simulink model "MyModel_Open_v1_1"  (R2018b)
settings: Solver=ode23tb  StartTime=0.0  StopTime=0.5  RelTol=1e-3
InitFcn:
  | Udc1 = 100;
  | Udc2 = 100;
  | tpwm = 1e-4;
  | Td = 0;
libraries: powerlib x33, powerlib_meascontrol x24, powerlib_extras x5, simulink x2
(part 1 of 2)
settings Model: Creator=chenhao  LastModifiedBy=chenhao

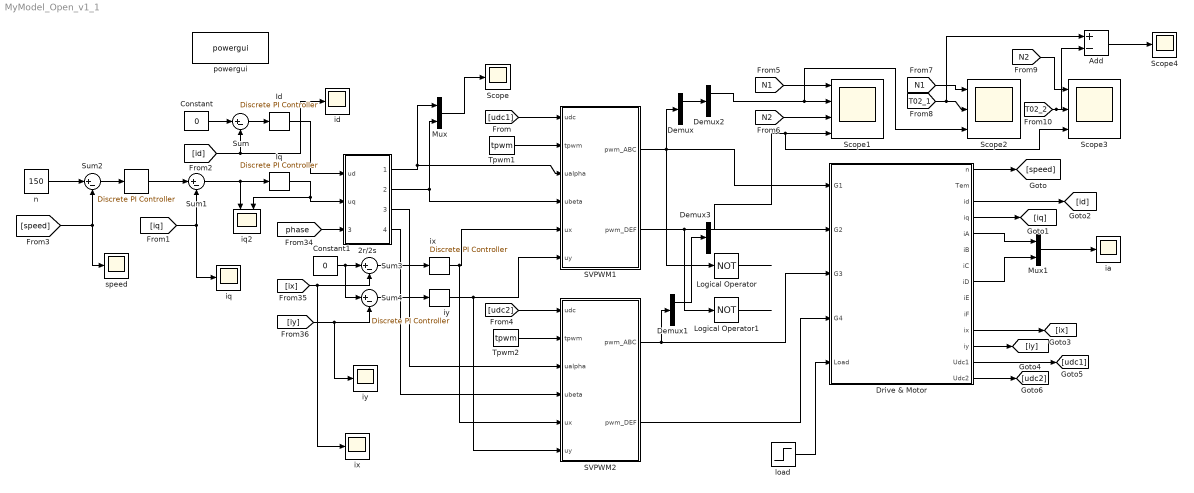
== system MyModel_Open_v1_1 ==
  "    " : powerlib_extras/Discrete  Control Blocks/Discrete PI Controller  Kp=1  Ki=80  Par_Limits=[50 -50]  Init=0  Ts=tpwm
  " Id" : powerlib_extras/Discrete  Control Blocks/Discrete PI Controller  Kp=3  Ki=120  Par_Limits=[300 -300]  Init=0  Ts=tpwm
  " Iq" : powerlib_extras/Discrete  Control Blocks/Discrete PI Controller  Kp=3  Ki=120  Par_Limits=[300 -300]  Init=0  Ts=tpwm
  " ix" : powerlib_extras/Discrete  Control Blocks/Discrete PI Controller  Kp=10  Ki=100  Par_Limits=[300 -300]  Init=0  Ts=tpwm
  " iy" : powerlib_extras/Discrete  Control Blocks/Discrete PI Controller  Kp=10  Ki=100  Par_Limits=[300 -300]  Init=0  Ts=tpwm
  2r/2s : Subsystem
  Add : Sum  Inputs=+-
  Constant : Constant  Value=0
  Constant1 : Constant  Value=0
  Demux : Demux  Outputs=3
  Demux1 : Demux  Outputs=3
  Demux2 : Demux  Outputs=2
  Demux3 : Demux  Outputs=2
  Drive & Motor : Subsystem
  Logical Operator : Logic  Operator=NOT  AllPortsSameDT=off  OutDataTypeStr=boolean
  Logical Operator1 : Logic  Operator=NOT  AllPortsSameDT=off  OutDataTypeStr=boolean
  Mux : Mux  Inputs=2
  Mux1 : Mux  Inputs=2
  SVPWM1 : Subsystem
  SVPWM2 : Subsystem
  Scope : Scope
  Scope1 : Scope  NumInputPorts=4
  Scope2 : Scope  NumInputPorts=3
  Scope3 : Scope  NumInputPorts=3
  Scope4 : Scope
  Sum{,1..4} (5 alike) : Sum  Inputs=|+-
  Tpwm1 : Constant  Value=tpwm
  Tpwm2 : Constant  Value=tpwm
  "ia " : Scope
  "id " : Scope
  iq : Scope
  iq2 : Scope  NumInputPorts=2
  ix : Scope
  iy : Scope
  load : Step  Time=0  After=15  SampleTime=0
  n : Constant  Value=150
  powergui : powerlib/powergui  Priority=1  SimulationMode=Discrete  SampleTime=5e-7  frequency=60  Iterations=50  frequencyindice=0  Pbase=100e6  ErrMax=1e-4  UnitsV=kV  UnitsW=MW  buscounter=0  FunctionMessages=off  echomessages=off  EnableUseOfTLC=off  CurrentSourceSwitches=off  DisableSnubberDevices=off  DisableRonSwitches=off  DisableVfSwitches=off  DisplayEquations=off  SolverType=Tustin/Backward Euler (TBE)  Interpol=off  ExternalGateDelay=off  methode=off  Ts=100  x0status=blocks  SPID=off  SwTol=0  HookPort=off  RestoreLinks=warning  ResistiveCurrentMeasurement=off  Frange=[0:2:500]  Ylog=off  Xlog=on  ShowGrid=off  save=off  variable=ZData  structure=Ia  ZoomFFT=on  StartTime=0.1  cycles=2  DisplayStyle=1  fundamental=2.5  FreqAxis=on  MaxFrequency=30  frequencyindicesteady=1  RmsSteady=1  display=off
  "speed " : Scope
  wires:
  2r/2s/2(ubeta1) -> SVPWM1/4(ubeta), Mux/2
  " ix"/1 -> SVPWM2/5(ux), SVPWM1/5(ux)
  Mux/1 -> Scope/1
  Tpwm1/1 -> SVPWM1/2(tpwm)
  load/1 -> Drive & Motor/5(Load)
  [iy] -> iy/1, Sum4/2
  [iq] -> iq/1, Sum1/2
  Sum3/1 -> " ix"/1
  [udc1] -> SVPWM1/1(udc)
  Sum2/1 -> "    "/1
  2r/2s/1(ualfa1) -> Mux/1, SVPWM1/3(ualpha)
  Sum1/1 -> iq2/1, " Iq"/1
  [speed] -> "speed "/1, Sum2/2
  Sum4/1 -> " iy"/1
  n/1 -> Sum2/1
  [ix] -> ix/1, Sum3/2
  " Id"/1 -> 2r/2s/1(ud)
  [phase] -> 2r/2s/3(theta)
  " Iq"/1 -> iq2/2, 2r/2s/2(uq)
  Sum/1 -> " Id"/1
  Constant1/1 -> Sum4/1, Sum3/1
  "    "/1 -> Sum1/1
  " iy"/1 -> SVPWM2/6(uy), SVPWM1/6(uy)
  [id] -> "id "/1, Sum/2
  Constant/1 -> Sum/1
  Drive & Motor/1(n) -> [speed]
  Drive & Motor/4(iq) -> [iq]
  Drive & Motor/3(id) -> [id]
  Drive & Motor/11(ix) -> [ix]
  Drive & Motor/12(iy) -> [iy]
  Drive & Motor/13(Udc1) -> [udc1]
  Drive & Motor/14(Udc2) -> [udc2]
  Drive & Motor/5(iA) -> Mux1/1
  Drive & Motor/8(iD) -> Mux1/2
  Mux1/1 -> "ia "/1
  [udc2] -> SVPWM2/1(udc)
  Tpwm2/1 -> SVPWM2/2(tpwm)
  2r/2s/3(ualfa2) -> SVPWM2/3(ualpha)
  2r/2s/4(ubeta2) -> SVPWM2/4(ubeta)
  SVPWM1/1(pwm_ABC) -> Demux/1, Logical Operator/1, Drive & Motor/1(G1)
  SVPWM1/2(pwm_DEF) -> Logical Operator1/1, Drive & Motor/2(G2)
  Logical Operator/1 -> ?
  SVPWM2/1(pwm_ABC) -> Demux1/1, Drive & Motor/3(G3)
  SVPWM2/2(pwm_DEF) -> Drive & Motor/4(G4)
  Logical Operator1/1 -> ?
  [N1] -> Scope1/1
  [N2] -> Scope1/3
  Demux/1 -> Demux2/1
  Demux2/1 -> Scope2/3, Scope1/2
  Demux1/1 -> Demux3/1
  Demux3/1 -> Scope3/3, Scope1/4
  [N1] -> Scope2/1
  [T02_1] -> Add/1, Scope2/2
  [N2] -> Scope3/1
  [T02_2] -> Add/2, Scope3/2
  Add/1 -> Scope4/1

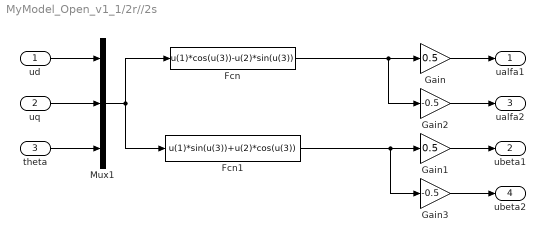
== system MyModel_Open_v1_1/2r//2s ==
  ud : Inport
  uq : Inport  Port=2
  theta : Inport  Port=3
  Fcn : Fcn  Expr=u(1)*cos(u(3))-u(2)*sin(u(3))
  Fcn1 : Fcn  Expr=u(1)*sin(u(3))+u(2)*cos(u(3))
  Gain : Gain  Gain=0.5
  Gain1 : Gain  Gain=0.5
  Gain2 : Gain  Gain=-0.5
  Gain3 : Gain  Gain=-0.5
  Mux1 : Mux  Inputs=3
  ualfa1 : Outport
  ubeta1 : Outport  Port=2
  ualfa2 : Outport  Port=3
  ubeta2 : Outport  Port=4
  wires:
  theta/1 -> Mux1/3
  uq/1 -> Mux1/2
  ud/1 -> Mux1/1
  Mux1/1 -> Fcn1/1, Fcn/1
  Fcn/1 -> Gain2/1, Gain/1
  Gain/1 -> ualfa1/1
  Gain1/1 -> ubeta1/1
  Fcn1/1 -> Gain3/1, Gain1/1
  Gain2/1 -> ualfa2/1
  Gain3/1 -> ubeta2/1

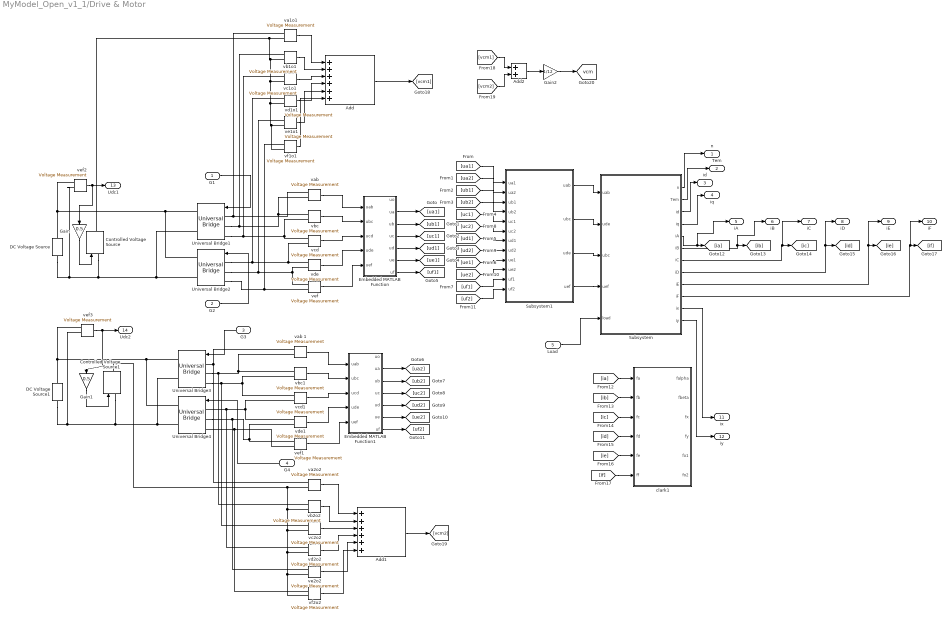
== system MyModel_Open_v1_1/Drive & Motor ==
  G1 : Inport
  G2 : Inport  Port=2
  G3 : Inport  Port=3
  G4 : Inport  Port=4
  Load : Inport  Port=5
  Add : Sum  Inputs=++++++
  Add1 : Sum  Inputs=++++++
  Add2 : Sum
  Controlled Voltage Source : powerlib/Electrical Sources/Controlled Voltage Source  Initialize=on  Source_Type=AC  Amplitude=0  Phase=0  Frequency=0  Measurements=None
  Controlled Voltage Source1 : powerlib/Electrical Sources/Controlled Voltage Source  Initialize=on  Source_Type=AC  Amplitude=0  Phase=0  Frequency=0  Measurements=None
  DC Voltage Source : powerlib/Electrical Sources/DC Voltage Source  Amplitude=Udc1  Measurements=Voltage
  DC Voltage Source1 : powerlib/Electrical Sources/DC Voltage Source  Amplitude=Udc2  Measurements=Voltage
  Embedded MATLAB Function : MATLAB Function  TreatAsAtomicUnit=on
  Embedded MATLAB Function1 : MATLAB Function  TreatAsAtomicUnit=on
  Gain : Gain  Gain=0.5
  Gain1 : Gain  Gain=0.5
  Gain2 : Gain  Gain=1/12
  Subsystem : Subsystem
  Subsystem1 : Subsystem
  Universal Bridge{1..4} (4 alike) : powerlib/Power Electronics/Universal Bridge  Arms=3  SnubberResistance=1e5  SnubberCapacitance=inf  Device=IGBT / Diodes  Ron=1e-3  Lon=0  ForwardVoltages="[  0  0  ]"  ForwardVoltage=0  GTOparameters=[ 10e-6 , 20e-6 ]  IGBTparameters=[ 0 , 0 ]  Measurements=None  Measurements_2=None  converterType=Rectifier
  clark1 : MATLAB Function  TreatAsAtomicUnit=on
  va1o1 : powerlib/Measurements/Voltage Measurement  PhasorSimulation=off  OutputType=Complex  PSBequivalent=0
  va2o2 : powerlib/Measurements/Voltage Measurement  PhasorSimulation=off  OutputType=Complex  PSBequivalent=0
  "vab " : powerlib/Measurements/Voltage Measurement  PhasorSimulation=off  OutputType=Complex  PSBequivalent=0
  vab 1 : powerlib/Measurements/Voltage Measurement  PhasorSimulation=off  OutputType=Complex  PSBequivalent=0
  vb1o1 : powerlib/Measurements/Voltage Measurement  PhasorSimulation=off  OutputType=Complex  PSBequivalent=0
  vb2o2 : powerlib/Measurements/Voltage Measurement  PhasorSimulation=off  OutputType=Complex  PSBequivalent=0
  vbc : powerlib/Measurements/Voltage Measurement  PhasorSimulation=off  OutputType=Complex  PSBequivalent=0
  vbc1 : powerlib/Measurements/Voltage Measurement  PhasorSimulation=off  OutputType=Complex  PSBequivalent=0
  vc1o1 : powerlib/Measurements/Voltage Measurement  PhasorSimulation=off  OutputType=Complex  PSBequivalent=0
  vc2o2 : powerlib/Measurements/Voltage Measurement  PhasorSimulation=off  OutputType=Complex  PSBequivalent=0
  vcd : powerlib/Measurements/Voltage Measurement  PhasorSimulation=off  OutputType=Complex  PSBequivalent=0
  vcd1 : powerlib/Measurements/Voltage Measurement  PhasorSimulation=off  OutputType=Complex  PSBequivalent=0
  vd1o1 : powerlib/Measurements/Voltage Measurement  PhasorSimulation=off  OutputType=Complex  PSBequivalent=0
  vd2o2 : powerlib/Measurements/Voltage Measurement  PhasorSimulation=off  OutputType=Complex  PSBequivalent=0
  vde : powerlib/Measurements/Voltage Measurement  PhasorSimulation=off  OutputType=Complex  PSBequivalent=0
  vde1 : powerlib/Measurements/Voltage Measurement  PhasorSimulation=off  OutputType=Complex  PSBequivalent=0
  ve1o1 : powerlib/Measurements/Voltage Measurement  PhasorSimulation=off  OutputType=Complex  PSBequivalent=0
  ve2o2 : powerlib/Measurements/Voltage Measurement  PhasorSimulation=off  OutputType=Complex  PSBequivalent=0
  vef{,1..3} (4 alike) : powerlib/Measurements/Voltage Measurement  PhasorSimulation=off  OutputType=Complex  PSBequivalent=0
  vf1o1 : powerlib/Measurements/Voltage Measurement  PhasorSimulation=off  OutputType=Complex  PSBequivalent=0
  vf2o2 : powerlib/Measurements/Voltage Measurement  PhasorSimulation=off  OutputType=Complex  PSBequivalent=0
  n : Outport
  Tem : Outport  Port=2
  id : Outport  Port=3
  iq : Outport  Port=4
  iA : Outport  Port=5
  iB : Outport  Port=6
  iC : Outport  Port=7
  iD : Outport  Port=8
  iE : Outport  Port=9
  iF : Outport  Port=10
  ix : Outport  Port=11
  iy : Outport  Port=12
  Udc1 : Outport  Port=13
  Udc2 : Outport  Port=14
  tag scope: vcm=global
  wires:
  G1/1 -> Universal Bridge1/1
  G2/1 -> Universal Bridge2/1
  G3/1 -> Universal Bridge3/1
  G4/1 -> Universal Bridge4/1
  vef/1 -> Embedded MATLAB Function/5(uef)
  vde/1 -> Embedded MATLAB Function/4(ude)
  "vab "/1 -> Embedded MATLAB Function/1(uab)
  vcd/1 -> Embedded MATLAB Function/3(ucd)
  vbc/1 -> Embedded MATLAB Function/2(ubc)
  Embedded MATLAB Function/2(ua) -> [ua1]
  Embedded MATLAB Function/3(ub) -> [ub1]
  Embedded MATLAB Function/4(uc) -> [uc1]
  Embedded MATLAB Function/5(ud) -> [ud1]
  Embedded MATLAB Function/6(ue) -> [ue1]
  Embedded MATLAB Function/7(uf) -> [uf1]
  Embedded MATLAB Function1/2(ua) -> [ua2]
  Embedded MATLAB Function1/3(ub) -> [ub2]
  Embedded MATLAB Function1/4(uc) -> [uc2]
  Embedded MATLAB Function1/5(ud) -> [ud2]
  Embedded MATLAB Function1/6(ue) -> [ue2]
  Embedded MATLAB Function1/7(uf) -> [uf2]
  vab 1/1 -> Embedded MATLAB Function1/1(uab)
  vbc1/1 -> Embedded MATLAB Function1/2(ubc)
  vcd1/1 -> Embedded MATLAB Function1/3(ucd)
  vde1/1 -> Embedded MATLAB Function1/4(ude)
  vef1/1 -> Embedded MATLAB Function1/5(uef)
  [ua1] -> Subsystem1/1(ua1)
  [ua2] -> Subsystem1/2(ua2)
  [ub1] -> Subsystem1/3(ub1)
  [ub2] -> Subsystem1/4(ub2)
  [uc1] -> Subsystem1/5(uc1)
  [uc2] -> Subsystem1/6(uc2)
  [ud1] -> Subsystem1/7(ud1)
  [ud2] -> Subsystem1/8(ud2)
  [ue1] -> Subsystem1/9(ue1)
  [ue2] -> Subsystem1/10(ue2)
  [uf1] -> Subsystem1/11(uf1)
  [uf2] -> Subsystem1/12(uf2)
  Load/1 -> Subsystem/5(load)
  Subsystem/1(n) -> n/1
  Subsystem/2(Tem) -> Tem/1
  Subsystem/3(id) -> id/1
  Subsystem/4(iq) -> iq/1
  Subsystem/5(iA) -> iA/1, [ia]
  Subsystem/6(iB) -> iB/1, [ib]
  Subsystem/7(iC) -> iC/1, [ic]
  Subsystem/8(iD) -> iD/1, [id]
  Subsystem/9(iE) -> iE/1, [ie]
  Subsystem/10(iF) -> iF/1, [if]
  [ia] -> clark1/1(fa)
  [ib] -> clark1/2(fb)
  [ic] -> clark1/3(fc)
  [id] -> clark1/4(fd)
  [ie] -> clark1/5(fe)
  [if] -> clark1/6(ff)
  vef2/1 -> Udc1/1, Gain/1
  vef3/1 -> Gain1/1, Udc2/1
  Gain/1 -> Controlled Voltage Source/1
  Gain1/1 -> Controlled Voltage Source1/1
  va1o1/1 -> Add/1
  vb1o1/1 -> Add/2
  vc1o1/1 -> Add/3
  vd1o1/1 -> Add/4
  ve1o1/1 -> Add/5
  vf1o1/1 -> Add/6
  Add/1 -> [vcm1]
  va2o2/1 -> Add1/1
  vb2o2/1 -> Add1/2
  vc2o2/1 -> Add1/3
  vd2o2/1 -> Add1/4
  ve2o2/1 -> Add1/5
  vf2o2/1 -> Add1/6
  Add1/1 -> [vcm2]
  [vcm1] -> Add2/1
  [vcm2] -> Add2/2
  Add2/1 -> Gain2/1
  Gain2/1 -> [vcm]
  Subsystem1/4(uef) -> Subsystem/4(uef)
  Subsystem1/3(ude) -> Subsystem/3(ubc)
  Subsystem1/2(ubc) -> Subsystem/2(ude)
  Subsystem1/1(uab) -> Subsystem/1(uab)
  Subsystem/11(ix) -> ix/1
  Subsystem/12(iy) -> iy/1
  connections:
  vde1/LConn1 -- vcd1/LConn2 -- vd2o2/LConn1 -- Universal Bridge4/LConn1
  vde/LConn1 -- vd1o1/LConn1 -- Universal Bridge2/LConn1 -- vcd/LConn2
  vef1/LConn2 -- Universal Bridge4/LConn3 -- vf2o2/LConn1
  Universal Bridge1/RConn2 -- Controlled Voltage Source/LConn1 -- vef2/LConn2 -- DC Voltage Source/LConn1 -- Universal Bridge2/RConn2
  DC Voltage Source/RConn1 -- Universal Bridge2/RConn1 -- Universal Bridge1/RConn1 -- vef2/LConn1
  Universal Bridge3/LConn1 -- vab 1/LConn1 -- va2o2/LConn1
  vbc/LConn1 -- vb1o1/LConn1 -- Universal Bridge1/LConn2 -- "vab "/LConn2
  vbc1/LConn1 -- vb2o2/LConn1 -- Universal Bridge3/LConn2 -- vab 1/LConn2
  vcd/LConn1 -- vc1o1/LConn1 -- Universal Bridge1/LConn3 -- vbc/LConn2
  vbc1/LConn2 -- vc2o2/LConn1 -- Universal Bridge3/LConn3 -- vcd1/LConn1
  Universal Bridge3/RConn1 -- vef3/LConn1 -- DC Voltage Source1/RConn1 -- Universal Bridge4/RConn1
  Universal Bridge3/RConn2 -- vef3/LConn2 -- DC Voltage Source1/LConn1 -- Controlled Voltage Source1/LConn1 -- Universal Bridge4/RConn2
  vef1/LConn1 -- ve2o2/LConn1 -- Universal Bridge4/LConn2 -- vde1/LConn2
  Universal Bridge1/LConn1 -- "vab "/LConn1 -- va1o1/LConn1
  vef/LConn1 -- ve1o1/LConn1 -- Universal Bridge2/LConn2 -- vde/LConn2
  Universal Bridge2/LConn3 -- vf1o1/LConn1 -- vef/LConn2
  va1o1/LConn2 -- vf1o1/LConn2 -- ve1o1/LConn2 -- vd1o1/LConn2 -- vc1o1/LConn2 -- vb1o1/LConn2 -- Controlled Voltage Source/RConn1
  va2o2/LConn2 -- vf2o2/LConn2 -- ve2o2/LConn2 -- vd2o2/LConn2 -- vc2o2/LConn2 -- vb2o2/LConn2 -- Controlled Voltage Source1/RConn1

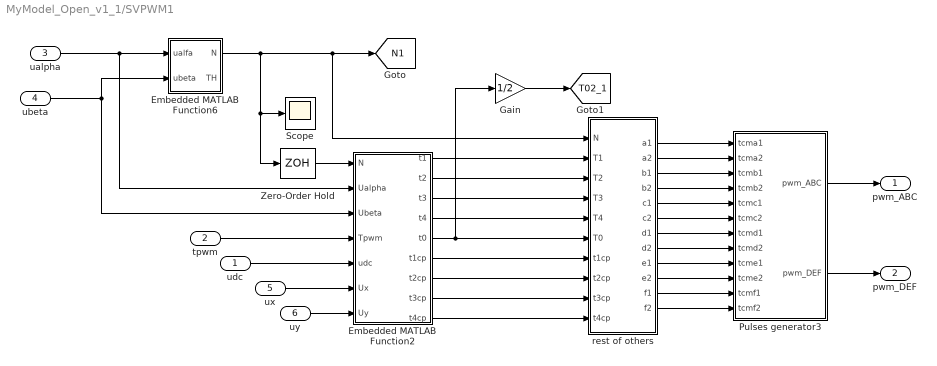
== system MyModel_Open_v1_1/SVPWM1 ==
  udc : Inport
  tpwm : Inport  Port=2
  ualpha : Inport  Port=3
  ubeta : Inport  Port=4
  ux : Inport  Port=5
  uy : Inport  Port=6
  Embedded MATLAB Function2 : MATLAB Function  TreatAsAtomicUnit=on
  Embedded MATLAB Function6 : MATLAB Function  TreatAsAtomicUnit=on
  Gain : Gain  Gain=1/2
  Pulses generator3 : Subsystem
  Scope : Scope
  Zero-Order Hold : ZeroOrderHold  SampleTime=1e-4
  rest of others : MATLAB Function  TreatAsAtomicUnit=on
  pwm_ABC : Outport
  pwm_DEF : Outport  Port=2
  tag scope: N1=global, T02_1=global
  wires:
  udc/1 -> Embedded MATLAB Function2/5(udc)
  Embedded MATLAB Function2/4(t4) -> rest of others/5(T4)
  Embedded MATLAB Function2/1(t1) -> rest of others/2(T1)
  Pulses generator3/1(pwm_ABC) -> pwm_ABC/1
  Pulses generator3/2(pwm_DEF) -> pwm_DEF/1
  rest of others/12(f2) -> Pulses generator3/12(tcmf2)
  rest of others/11(f1) -> Pulses generator3/11(tcmf1)
  rest of others/10(e2) -> Pulses generator3/10(tcme2)
  rest of others/9(e1) -> Pulses generator3/9(tcme1)
  rest of others/8(d2) -> Pulses generator3/8(tcmd2)
  rest of others/7(d1) -> Pulses generator3/7(tcmd1)
  rest of others/6(c2) -> Pulses generator3/6(tcmc2)
  rest of others/5(c1) -> Pulses generator3/5(tcmc1)
  rest of others/4(b2) -> Pulses generator3/4(tcmb2)
  rest of others/3(b1) -> Pulses generator3/3(tcmb1)
  rest of others/2(a2) -> Pulses generator3/2(tcma2)
  rest of others/1(a1) -> Pulses generator3/1(tcma1)
  Embedded MATLAB Function2/2(t2) -> rest of others/3(T2)
  tpwm/1 -> Embedded MATLAB Function2/4(Tpwm)
  Embedded MATLAB Function2/5(t0) -> Gain/1, rest of others/6(T0)
  ualpha/1 -> Embedded MATLAB Function2/2(Ualpha), Embedded MATLAB Function6/1(ualfa)
  ubeta/1 -> Embedded MATLAB Function6/2(ubeta), Embedded MATLAB Function2/3(Ubeta)
  ux/1 -> Embedded MATLAB Function2/6(Ux)
  uy/1 -> Embedded MATLAB Function2/7(Uy)
  Embedded MATLAB Function2/3(t3) -> rest of others/4(T3)
  Zero-Order Hold/1 -> Embedded MATLAB Function2/1(N)
  Embedded MATLAB Function6/1(N) -> [N1], rest of others/1(N), Scope/1, Zero-Order Hold/1
  Embedded MATLAB Function2/9(t4cp) -> rest of others/10(t4cp)
  Embedded MATLAB Function2/8(t3cp) -> rest of others/9(t3cp)
  Embedded MATLAB Function2/7(t2cp) -> rest of others/8(t2cp)
  Embedded MATLAB Function2/6(t1cp) -> rest of others/7(t1cp)
  Gain/1 -> [T02_1]

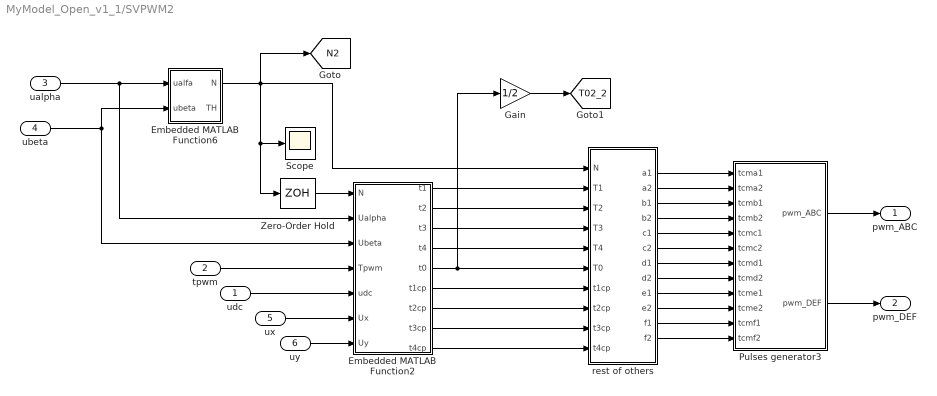
== system MyModel_Open_v1_1/SVPWM2 ==
  udc : Inport
  tpwm : Inport  Port=2
  ualpha : Inport  Port=3
  ubeta : Inport  Port=4
  ux : Inport  Port=5
  uy : Inport  Port=6
  Embedded MATLAB Function2 : MATLAB Function  TreatAsAtomicUnit=on
  Embedded MATLAB Function6 : MATLAB Function  TreatAsAtomicUnit=on
  Gain : Gain  Gain=1/2
  Pulses generator3 : Subsystem
  Scope : Scope
  Zero-Order Hold : ZeroOrderHold  SampleTime=1e-4
  rest of others : MATLAB Function  TreatAsAtomicUnit=on
  pwm_ABC : Outport
  pwm_DEF : Outport  Port=2
  tag scope: N2=global, T02_2=global
  wires:
  Embedded MATLAB Function2/6(t1cp) -> rest of others/7(t1cp)
  Embedded MATLAB Function2/7(t2cp) -> rest of others/8(t2cp)
  Embedded MATLAB Function2/8(t3cp) -> rest of others/9(t3cp)
  Embedded MATLAB Function2/9(t4cp) -> rest of others/10(t4cp)
  Embedded MATLAB Function6/1(N) -> Zero-Order Hold/1, Scope/1, rest of others/1(N), [N2]
  Zero-Order Hold/1 -> Embedded MATLAB Function2/1(N)
  Embedded MATLAB Function2/3(t3) -> rest of others/4(T3)
  uy/1 -> Embedded MATLAB Function2/7(Uy)
  ux/1 -> Embedded MATLAB Function2/6(Ux)
  ubeta/1 -> Embedded MATLAB Function2/3(Ubeta), Embedded MATLAB Function6/2(ubeta)
  ualpha/1 -> Embedded MATLAB Function6/1(ualfa), Embedded MATLAB Function2/2(Ualpha)
  Embedded MATLAB Function2/5(t0) -> Gain/1, rest of others/6(T0)
  tpwm/1 -> Embedded MATLAB Function2/4(Tpwm)
  Embedded MATLAB Function2/2(t2) -> rest of others/3(T2)
  rest of others/1(a1) -> Pulses generator3/1(tcma1)
  rest of others/2(a2) -> Pulses generator3/2(tcma2)
  rest of others/3(b1) -> Pulses generator3/3(tcmb1)
  rest of others/4(b2) -> Pulses generator3/4(tcmb2)
  rest of others/5(c1) -> Pulses generator3/5(tcmc1)
  rest of others/6(c2) -> Pulses generator3/6(tcmc2)
  rest of others/7(d1) -> Pulses generator3/7(tcmd1)
  rest of others/8(d2) -> Pulses generator3/8(tcmd2)
  rest of others/9(e1) -> Pulses generator3/9(tcme1)
  rest of others/10(e2) -> Pulses generator3/10(tcme2)
  rest of others/11(f1) -> Pulses generator3/11(tcmf1)
  rest of others/12(f2) -> Pulses generator3/12(tcmf2)
  Pulses generator3/2(pwm_DEF) -> pwm_DEF/1
  Pulses generator3/1(pwm_ABC) -> pwm_ABC/1
  Embedded MATLAB Function2/1(t1) -> rest of others/2(T1)
  Embedded MATLAB Function2/4(t4) -> rest of others/5(T4)
  udc/1 -> Embedded MATLAB Function2/5(udc)
  Gain/1 -> [T02_2]

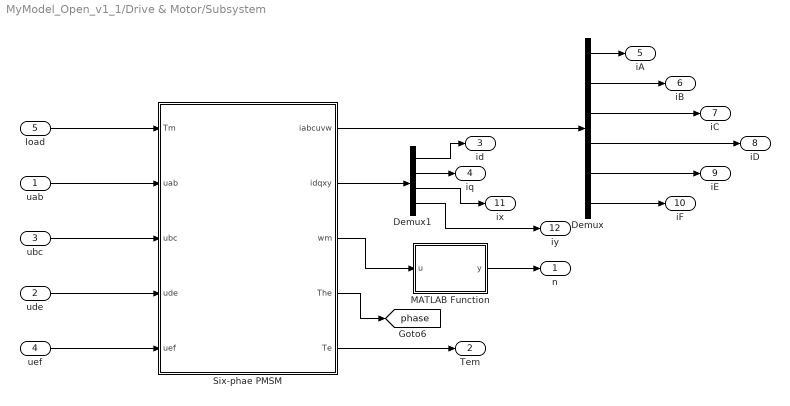
== system MyModel_Open_v1_1/Drive & Motor/Subsystem ==
  uab : Inport
  ude : Inport  Port=2
  ubc : Inport  Port=3
  uef : Inport  Port=4
  load : Inport  Port=5
  Demux : Demux  Outputs=6
  Demux1 : Demux
  MATLAB Function : MATLAB Function  TreatAsAtomicUnit=on
  Six-phae PMSM : Subsystem  mask{R=0.099, Ld=2.463342136542000e-03, Lq=2.473254136542000e-03, Lz=1.520747e-3, Flux=0.0592, J=0.00174, F=0, p=5}
      mask prompts: R "R(ohm)"; Ld "Ld(H)"; Lq "Lq(H)"; Lz "Lz(H)"; Flux "Flux(Wb)"; J "J(kg.m^2)"; F "F(N.m.s)"
  n : Outport
  Tem : Outport  Port=2
  id : Outport  Port=3
  iq : Outport  Port=4
  iA : Outport  Port=5
  iB : Outport  Port=6
  iC : Outport  Port=7
  iD : Outport  Port=8
  iE : Outport  Port=9
  iF : Outport  Port=10
  ix : Outport  Port=11
  iy : Outport  Port=12
  tag scope: phase=global
  wires:
  Demux/6 -> iF/1
  Demux1/2 -> iq/1
  uef/1 -> Six-phae PMSM/5(uef)
  Demux/5 -> iE/1
  Demux/2 -> iB/1
  Demux/1 -> iA/1
  Six-phae PMSM/5(Te) -> Tem/1
  uab/1 -> Six-phae PMSM/2(uab)
  Demux1/1 -> id/1
  ubc/1 -> Six-phae PMSM/3(ubc)
  Demux/3 -> iC/1
  MATLAB Function/1(y) -> n/1
  load/1 -> Six-phae PMSM/1(Tm)
  Demux/4 -> iD/1
  ude/1 -> Six-phae PMSM/4(ude)
  Six-phae PMSM/1(iabcuvw) -> Demux/1
  Six-phae PMSM/2(idqxy) -> Demux1/1
  Demux1/3 -> ix/1
  Demux1/4 -> iy/1
  Six-phae PMSM/3(wm) -> MATLAB Function/1(u)
  Six-phae PMSM/4(The) -> [phase]

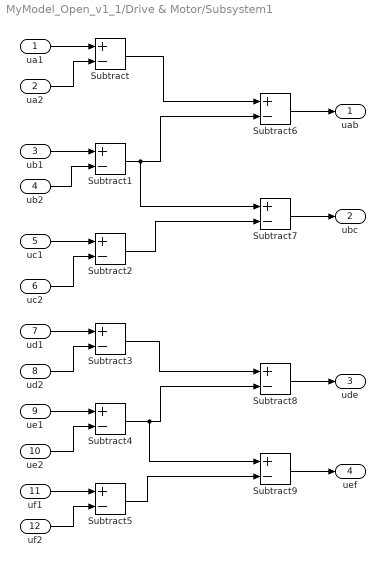
== system MyModel_Open_v1_1/Drive & Motor/Subsystem1 ==
  ua1 : Inport
  ua2 : Inport  Port=2
  ub1 : Inport  Port=3
  ub2 : Inport  Port=4
  uc1 : Inport  Port=5
  uc2 : Inport  Port=6
  ud1 : Inport  Port=7
  ud2 : Inport  Port=8
  ue1 : Inport  Port=9
  ue2 : Inport  Port=10
  uf1 : Inport  Port=11
  uf2 : Inport  Port=12
  Subtract{,1..9} (10 alike) : Sum  Inputs=+-
  uab : Outport
  ubc : Outport  Port=2
  ude : Outport  Port=3
  uef : Outport  Port=4
  wires:
  ua1/1 -> Subtract/1
  ua2/1 -> Subtract/2
  Subtract/1 -> Subtract6/1
  ub1/1 -> Subtract1/1
  ub2/1 -> Subtract1/2
  Subtract1/1 -> Subtract7/1, Subtract6/2
  uc1/1 -> Subtract2/1
  uc2/1 -> Subtract2/2
  Subtract2/1 -> Subtract7/2
  ud1/1 -> Subtract3/1
  ud2/1 -> Subtract3/2
  Subtract3/1 -> Subtract8/1
  ue1/1 -> Subtract4/1
  ue2/1 -> Subtract4/2
  Subtract4/1 -> Subtract9/1, Subtract8/2
  uf1/1 -> Subtract5/1
  uf2/1 -> Subtract5/2
  Subtract5/1 -> Subtract9/2
  Subtract6/1 -> uab/1
  Subtract7/1 -> ubc/1
  Subtract8/1 -> ude/1
  Subtract9/1 -> uef/1

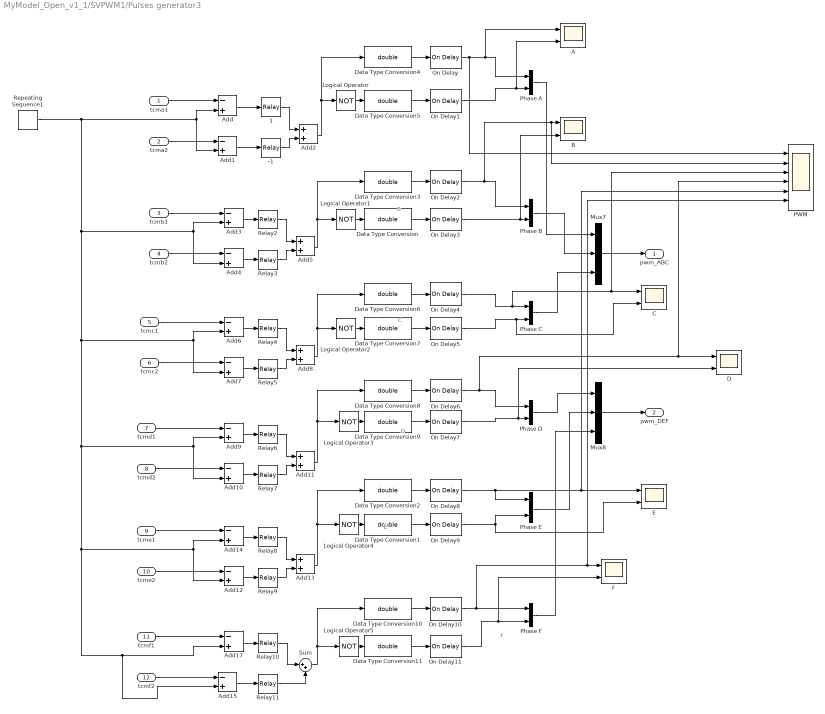
== system MyModel_Open_v1_1/SVPWM1/Pulses generator3 ==
  note: B
  note: C
  note: D
  note: E
  note: F
  tcma1 : Inport
  tcma2 : Inport  Port=2
  tcmb1 : Inport  Port=3
  tcmb2 : Inport  Port=4
  tcmc1 : Inport  Port=5
  tcmc2 : Inport  Port=6
  tcmd1 : Inport  Port=7
  tcmd2 : Inport  Port=8
  tcme1 : Inport  Port=9
  tcme2 : Inport  Port=10
  tcmf1 : Inport  Port=11
  tcmf2 : Inport  Port=12
  -1 : Relay  OnOutputValue=-1
  1 : Relay
  A : Scope  NumInputPorts=2
  Add{,1,3..4,6..7,9..10,12,14..15,17} (12 alike) : Sum  Inputs=-+
  Add{2,5,8,11,13} (5 alike) : Sum
  B : Scope  NumInputPorts=2
  C : Scope  NumInputPorts=2
  D : Scope  NumInputPorts=2
  Data Type Conversion{,1..11} (12 alike) : DataTypeConversion  OutDataTypeStr=double
  E : Scope  NumInputPorts=2
  F : Scope  NumInputPorts=2
  Logical Operator{,1..5} (6 alike) : Logic  Operator=NOT  AllPortsSameDT=off  OutDataTypeStr=boolean
  Mux7 : Mux  Inputs=3
  Mux8 : Mux  Inputs=3
  On Delay{,1..11} (12 alike) : powerlib_meascontrol/Logic/On Delay  DelayType=On delay  delay=Td  ic=0  Ts=0
      settings: SourceProductName=Simscape Power Systems
  PWM : Scope  NumInputPorts=6
  Phase A : Mux  Inputs=2
  Phase B : Mux  Inputs=2
  Phase C : Mux  Inputs=2
  Phase D : Mux  Inputs=2
  Phase E : Mux  Inputs=2
  Phase F : Mux  Inputs=2
  Relay{2,4,6,8,10} (5 alike) : Relay
  Relay{3,5,7,9,11} (5 alike) : Relay  OnOutputValue=-1
  Repeating Sequence1 : simulink/Sources/Repeating Sequence  rep_seq_t=[0 tpwm]  rep_seq_y=[0 tpwm]
  Sum : Sum  Inputs=|++
  pwm_ABC : Outport
  pwm_DEF : Outport  Port=2
  wires:
  On Delay11/1 -> F/2, Phase F/2
  Data Type Conversion11/1 -> On Delay11/1
  On Delay10/1 -> PWM/6, F/1, Phase F/1
  Data Type Conversion10/1 -> On Delay10/1
  On Delay9/1 -> E/2, Phase E/2
  Data Type Conversion1/1 -> On Delay9/1
  On Delay8/1 -> Phase E/1, PWM/5, E/1
  Data Type Conversion2/1 -> On Delay8/1
  On Delay7/1 -> D/2, Phase D/2
  Data Type Conversion9/1 -> On Delay7/1
  On Delay6/1 -> PWM/4, D/1, Phase D/1
  Data Type Conversion8/1 -> On Delay6/1
  On Delay5/1 -> C/2, Phase C/2
  Data Type Conversion7/1 -> On Delay5/1
  On Delay4/1 -> PWM/3, C/1, Phase C/1
  Data Type Conversion6/1 -> On Delay4/1
  On Delay2/1 -> PWM/2, B/1, Phase B/1
  On Delay3/1 -> B/2, Phase B/2
  Data Type Conversion/1 -> On Delay3/1
  Data Type Conversion3/1 -> On Delay2/1
  On Delay1/1 -> A/2, Phase A/2
  Data Type Conversion5/1 -> On Delay1/1
  On Delay/1 -> A/1, Phase A/1, PWM/1
  Data Type Conversion4/1 -> On Delay/1
  Logical Operator3/1 -> Data Type Conversion9/1
  Logical Operator2/1 -> Data Type Conversion7/1
  Logical Operator/1 -> Data Type Conversion5/1
  Logical Operator1/1 -> Data Type Conversion/1
  Logical Operator4/1 -> Data Type Conversion1/1
  Add5/1 -> Logical Operator1/1, Data Type Conversion3/1
  Add2/1 -> Logical Operator/1, Data Type Conversion4/1
  Mux8/1 -> pwm_DEF/1
  Mux7/1 -> pwm_ABC/1
  Sum/1 -> Logical Operator5/1, Data Type Conversion10/1
  Add13/1 -> Logical Operator4/1, Data Type Conversion2/1
  Add11/1 -> Logical Operator3/1, Data Type Conversion8/1
  Add8/1 -> Logical Operator2/1, Data Type Conversion6/1
  Logical Operator5/1 -> Data Type Conversion11/1
  tcmf2/1 -> Add15/1
  Relay11/1 -> Sum/2
  Relay10/1 -> Sum/1
  Add17/1 -> Relay10/1
  tcmf1/1 -> Add17/1
  tcme2/1 -> Add12/1
  Relay9/1 -> Add13/2
  Relay8/1 -> Add13/1
  Add12/1 -> Relay9/1
  Add14/1 -> Relay8/1
  tcme1/1 -> Add14/1
  tcmd2/1 -> Add10/1
  Relay7/1 -> Add11/2
  Relay6/1 -> Add11/1
  Add10/1 -> Relay7/1
  Add9/1 -> Relay6/1
  tcmd1/1 -> Add9/1
  tcmc2/1 -> Add7/1
  Relay5/1 -> Add8/2
  Relay4/1 -> Add8/1
  Add7/1 -> Relay5/1
  Add6/1 -> Relay4/1
  tcmb2/1 -> Add4/1
  Relay3/1 -> Add5/2
  Relay2/1 -> Add5/1
  Add4/1 -> Relay3/1
  Add3/1 -> Relay2/1
  tcma1/1 -> Add/1
  -1/1 -> Add2/2
  1/1 -> Add2/1
  Add1/1 -> -1/1
  Add/1 -> 1/1
  Repeating Sequence1/1 -> Add15/2, Add17/2, Add12/2, Add14/2, Add9/2, Add10/2, Add7/2, Add6/2, Add3/2, Add4/2, Add1/2, Add/2
  tcma2/1 -> Add1/1
  tcmb1/1 -> Add3/1
  tcmc1/1 -> Add6/1
  Add15/1 -> Relay11/1
  Phase A/1 -> Mux7/1
  Phase B/1 -> Mux7/2
  Phase C/1 -> Mux7/3
  Phase D/1 -> Mux8/1
  Phase E/1 -> Mux8/2
  Phase F/1 -> Mux8/3

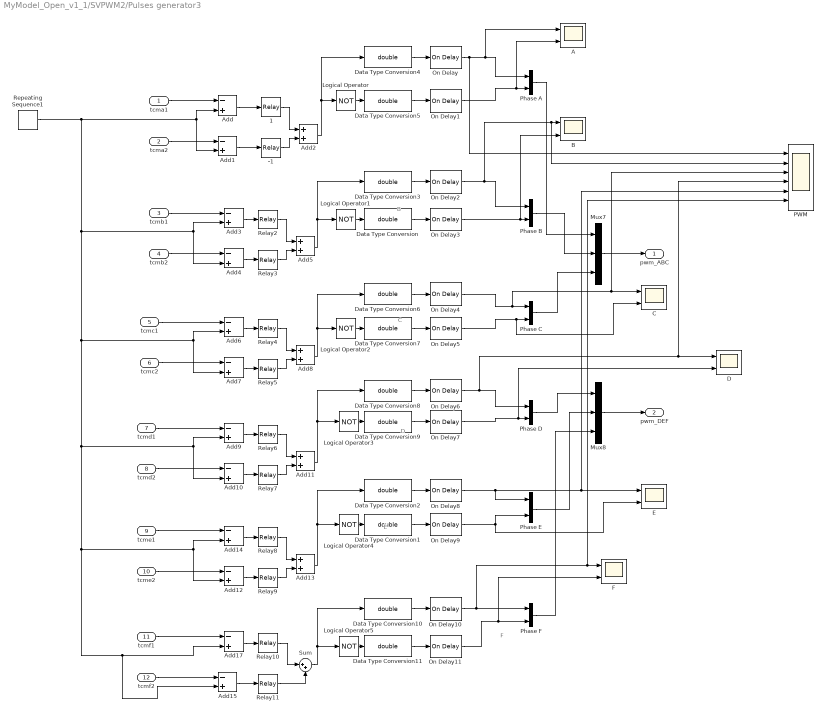
== system MyModel_Open_v1_1/SVPWM2/Pulses generator3 ==
  note: F
  note: E
  note: D
  note: C
  note: B
  tcma1 : Inport
  tcma2 : Inport  Port=2
  tcmb1 : Inport  Port=3
  tcmb2 : Inport  Port=4
  tcmc1 : Inport  Port=5
  tcmc2 : Inport  Port=6
  tcmd1 : Inport  Port=7
  tcmd2 : Inport  Port=8
  tcme1 : Inport  Port=9
  tcme2 : Inport  Port=10
  tcmf1 : Inport  Port=11
  tcmf2 : Inport  Port=12
  -1 : Relay  OnOutputValue=-1
  1 : Relay
  A : Scope  NumInputPorts=2
  Add{,1,3..4,6..7,9..10,12,14..15,17} (12 alike) : Sum  Inputs=-+
  Add{2,5,8,11,13} (5 alike) : Sum
  B : Scope  NumInputPorts=2
  C : Scope  NumInputPorts=2
  D : Scope  NumInputPorts=2
  Data Type Conversion{,1..11} (12 alike) : DataTypeConversion  OutDataTypeStr=double
  E : Scope  NumInputPorts=2
  F : Scope  NumInputPorts=2
  Logical Operator{,1..5} (6 alike) : Logic  Operator=NOT  AllPortsSameDT=off  OutDataTypeStr=boolean
  Mux7 : Mux  Inputs=3
  Mux8 : Mux  Inputs=3
  On Delay{,1..11} (12 alike) : powerlib_meascontrol/Logic/On Delay  DelayType=On delay  delay=Td  ic=0  Ts=0
      settings: SourceProductName=Simscape Power Systems
  PWM : Scope  NumInputPorts=6
  Phase A : Mux  Inputs=2
  Phase B : Mux  Inputs=2
  Phase C : Mux  Inputs=2
  Phase D : Mux  Inputs=2
  Phase E : Mux  Inputs=2
  Phase F : Mux  Inputs=2
  Relay{2,4,6,8,10} (5 alike) : Relay
  Relay{3,5,7,9,11} (5 alike) : Relay  OnOutputValue=-1
  Repeating Sequence1 : simulink/Sources/Repeating Sequence  rep_seq_t=[0 tpwm]  rep_seq_y=[0 tpwm]
  Sum : Sum  Inputs=|++
  pwm_ABC : Outport
  pwm_DEF : Outport  Port=2
  wires:
  Phase F/1 -> Mux8/3
  Phase E/1 -> Mux8/2
  Phase D/1 -> Mux8/1
  Phase C/1 -> Mux7/3
  Phase B/1 -> Mux7/2
  Phase A/1 -> Mux7/1
  Add15/1 -> Relay11/1
  tcmc1/1 -> Add6/1
  tcmb1/1 -> Add3/1
  tcma2/1 -> Add1/1
  Repeating Sequence1/1 -> Add/2, Add1/2, Add4/2, Add3/2, Add6/2, Add7/2, Add10/2, Add9/2, Add14/2, Add12/2, Add17/2, Add15/2
  Add/1 -> 1/1
  Add1/1 -> -1/1
  1/1 -> Add2/1
  -1/1 -> Add2/2
  tcma1/1 -> Add/1
  Add3/1 -> Relay2/1
  Add4/1 -> Relay3/1
  Relay2/1 -> Add5/1
  Relay3/1 -> Add5/2
  tcmb2/1 -> Add4/1
  Add6/1 -> Relay4/1
  Add7/1 -> Relay5/1
  Relay4/1 -> Add8/1
  Relay5/1 -> Add8/2
  tcmc2/1 -> Add7/1
  tcmd1/1 -> Add9/1
  Add9/1 -> Relay6/1
  Add10/1 -> Relay7/1
  Relay6/1 -> Add11/1
  Relay7/1 -> Add11/2
  tcmd2/1 -> Add10/1
  tcme1/1 -> Add14/1
  Add14/1 -> Relay8/1
  Add12/1 -> Relay9/1
  Relay8/1 -> Add13/1
  Relay9/1 -> Add13/2
  tcme2/1 -> Add12/1
  tcmf1/1 -> Add17/1
  Add17/1 -> Relay10/1
  Relay10/1 -> Sum/1
  Relay11/1 -> Sum/2
  tcmf2/1 -> Add15/1
  Logical Operator5/1 -> Data Type Conversion11/1
  Add8/1 -> Data Type Conversion6/1, Logical Operator2/1
  Add11/1 -> Data Type Conversion8/1, Logical Operator3/1
  Add13/1 -> Data Type Conversion2/1, Logical Operator4/1
  Sum/1 -> Data Type Conversion10/1, Logical Operator5/1
  Mux7/1 -> pwm_ABC/1
  Mux8/1 -> pwm_DEF/1
  Add2/1 -> Data Type Conversion4/1, Logical Operator/1
  Add5/1 -> Data Type Conversion3/1, Logical Operator1/1
  Logical Operator4/1 -> Data Type Conversion1/1
  Logical Operator1/1 -> Data Type Conversion/1
  Logical Operator/1 -> Data Type Conversion5/1
  Logical Operator2/1 -> Data Type Conversion7/1
  Logical Operator3/1 -> Data Type Conversion9/1
  Data Type Conversion4/1 -> On Delay/1
  On Delay/1 -> PWM/1, Phase A/1, A/1
  Data Type Conversion5/1 -> On Delay1/1
  On Delay1/1 -> Phase A/2, A/2
  Data Type Conversion3/1 -> On Delay2/1
  Data Type Conversion/1 -> On Delay3/1
  On Delay3/1 -> Phase B/2, B/2
  On Delay2/1 -> Phase B/1, B/1, PWM/2
  Data Type Conversion6/1 -> On Delay4/1
  On Delay4/1 -> Phase C/1, C/1, PWM/3
  Data Type Conversion7/1 -> On Delay5/1
  On Delay5/1 -> Phase C/2, C/2
  Data Type Conversion8/1 -> On Delay6/1
  On Delay6/1 -> Phase D/1, D/1, PWM/4
  Data Type Conversion9/1 -> On Delay7/1
  On Delay7/1 -> Phase D/2, D/2
  Data Type Conversion2/1 -> On Delay8/1
  On Delay8/1 -> E/1, PWM/5, Phase E/1
  Data Type Conversion1/1 -> On Delay9/1
  On Delay9/1 -> Phase E/2, E/2
  Data Type Conversion10/1 -> On Delay10/1
  On Delay10/1 -> Phase F/1, F/1, PWM/6
  Data Type Conversion11/1 -> On Delay11/1
  On Delay11/1 -> Phase F/2, F/2

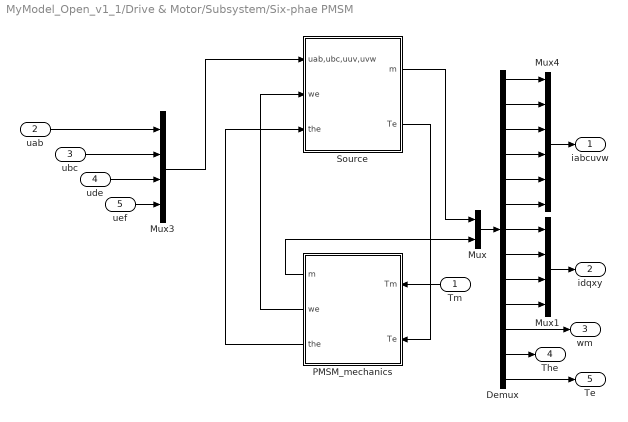
== system MyModel_Open_v1_1/Drive & Motor/Subsystem/Six-phae PMSM ==
  Tm : Inport
  uab : Inport  Port=2
  ubc : Inport  Port=3
  ude : Inport  Port=4
  uef : Inport  Port=5
  Demux : Demux  Outputs=13
  Mux : Mux  Inputs=2
  Mux1 : Mux
  Mux3 : Mux
  Mux4 : Mux  Inputs=6
  PMSM_mechanics : Subsystem
  Source : Subsystem
  iabcuvw : Outport
  idqxy : Outport  Port=2
  wm : Outport  Port=3
  The : Outport  Port=4
  Te : Outport  Port=5
  wires:
  Tm/1 -> PMSM_mechanics/1(Tm)
  Source/2(Te) -> PMSM_mechanics/2(Te)
  PMSM_mechanics/2(we) -> Source/2(we)
  PMSM_mechanics/3(the) -> Source/3(the)
  PMSM_mechanics/1(m) -> Mux/2
  Source/1(m) -> Mux/1
  Mux3/1 -> Source/1(uab,ubc,uuv,uvw)
  Mux/1 -> Demux/1
  Mux4/1 -> iabcuvw/1
  Mux1/1 -> idqxy/1
  Demux/12 -> The/1
  Demux/13 -> Te/1
  Demux/5 -> Mux4/5
  Demux/2 -> Mux4/2
  Demux/3 -> Mux4/3
  Demux/6 -> Mux4/6
  Demux/4 -> Mux4/4
  Demux/1 -> Mux4/1
  Demux/7 -> Mux1/1
  Demux/8 -> Mux1/2
  Demux/9 -> Mux1/3
  Demux/10 -> Mux1/4
  Demux/11 -> wm/1
  uab/1 -> Mux3/1
  ubc/1 -> Mux3/2
  ude/1 -> Mux3/3
  uef/1 -> Mux3/4

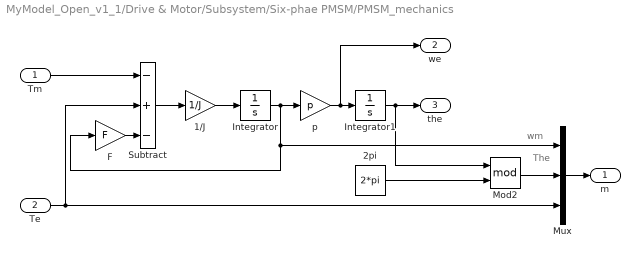
== system MyModel_Open_v1_1/Drive & Motor/Subsystem/Six-phae PMSM/PMSM_mechanics ==
  note: The
  note: wm
  Tm : Inport
  Te : Inport  Port=2
  1/J : Gain  Gain=1/J
  2pi : Constant  Value=2*pi
  F : Gain  Gain=F
  Integrator : Integrator
  Integrator1 : Integrator
  Mod2 : Math  Operator=mod  SaturateOnIntegerOverflow=on
  Mux : Mux  Inputs=3
  Subtract : Sum  Inputs=-+-
  p : Gain  Gain=p
  m : Outport
  we : Outport  Port=2
  the : Outport  Port=3
  wires:
  Tm/1 -> Subtract/1
  Te/1 -> Subtract/2, Mux/3
  Subtract/1 -> 1/J/1
  1/J/1 -> Integrator/1
  Integrator/1 -> p/1, F/1, Mux/1
  F/1 -> Subtract/3
  p/1 -> Integrator1/1, we/1
  Integrator1/1 -> the/1, Mod2/1
  Mux/1 -> m/1
  Mod2/1 -> Mux/2
  2pi/1 -> Mod2/2

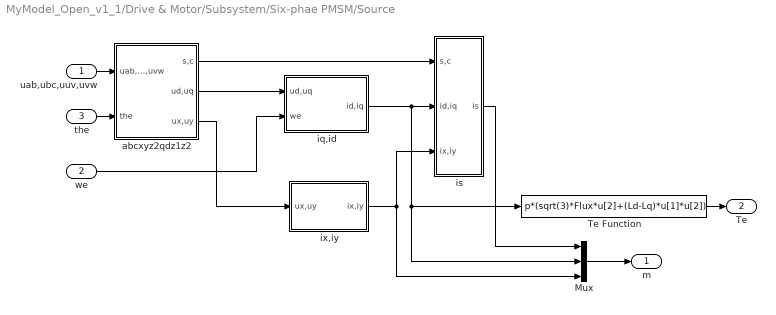
== system MyModel_Open_v1_1/Drive & Motor/Subsystem/Six-phae PMSM/Source ==
  uab,ubc,uuv,uvw : Inport
  we : Inport  Port=2
  the : Inport  Port=3
  Mux : Mux  Inputs=3
  Te Function : Fcn  Expr=p*(sqrt(3)*Flux*u[2]+(Ld-Lq)*u[1]*u[2])
  abcxyz2qdz1z2 : Subsystem
  iq,id : Subsystem
  is : Subsystem
  ix,iy : Subsystem
  m : Outport
  Te : Outport  Port=2
  wires:
  uab,ubc,uuv,uvw/1 -> abcxyz2qdz1z2/1(uab,ubc,uuv,uvw)
  the/1 -> abcxyz2qdz1z2/2(the)
  abcxyz2qdz1z2/2(ud,uq) -> iq,id/1(ud,uq)
  we/1 -> iq,id/2(we)
  abcxyz2qdz1z2/1(s,c) -> is/1(s,c)
  iq,id/1(id,iq) -> is/2(id,iq), Mux/2, Te Function/1
  Te Function/1 -> Te/1
  abcxyz2qdz1z2/3(ux,uy) -> ix,iy/1(ux,uy)
  ix,iy/1(ix,iy) -> is/3(ix,iy), Mux/3
  Mux/1 -> m/1
  is/1(is) -> Mux/1

== system MyModel_Open_v1_1/Drive & Motor/Subsystem/Six-phae PMSM/Source/abcxyz2qdz1z2 ==
  uab,ubc,uuv,uvw : Inport
  the : Inport  Port=2
  Clarke : Subsystem
  Mux2 : Mux  Inputs=2
  PARK : Subsystem
  Trigonometric Function : Trigonometry
  Trigonometric Function1 : Trigonometry  Operator=cos
  s,c : Outport
  ud,uq : Outport  Port=2
  ux,uy : Outport  Port=3
  wires:
  Mux2/1 -> PARK/2(s,c), s,c/1
  the/1 -> Trigonometric Function1/1, Trigonometric Function/1
  PARK/1(ud,uq) -> ud,uq/1
  uab,ubc,uuv,uvw/1 -> Clarke/1(uab,ubc,uuv,uvw)
  Trigonometric Function1/1 -> Mux2/2
  Trigonometric Function/1 -> Mux2/1
  Clarke/1(ualpha,ubeta) -> PARK/1(ualpha,ubeta)
  Clarke/2(ux,uy) -> ux,uy/1

== system MyModel_Open_v1_1/Drive & Motor/Subsystem/Six-phae PMSM/Source/iq,id ==
  ud,uq : Inport
  we : Inport  Port=2
  Demux : Demux  Outputs=2
  Mux : Mux  Inputs=2
  id : Subsystem
  iq : Subsystem
  id,iq : Outport
  wires:
  ud,uq/1 -> Demux/1
  Mux/1 -> id,iq/1
  Demux/1 -> id/1(ud)
  Demux/2 -> iq/3(uq)
  we/1 -> iq/2(we), id/2(we)
  iq/1(iq) -> id/3(iq), Mux/2
  id/1(id) -> iq/1(id), Mux/1

== system MyModel_Open_v1_1/Drive & Motor/Subsystem/Six-phae PMSM/Source/is ==
  s,c : Inport
  id,iq : Inport  Port=2
  ix,iy : Inport  Port=3
  IClarke : Subsystem
  IPARK : Subsystem
  is : Outport
  wires:
  s,c/1 -> IPARK/1(s,c)
  id,iq/1 -> IPARK/2(id,iq)
  IPARK/1(ialpha,ibeta) -> IClarke/1(ialpha,ibeta)
  ix,iy/1 -> IClarke/2(ix,iy)
  IClarke/1(iabcuvw) -> is/1

== system MyModel_Open_v1_1/Drive & Motor/Subsystem/Six-phae PMSM/Source/ix,iy ==
  ux,uy : Inport
  Demux : Demux  Outputs=2
  Mux : Mux  Inputs=2
  ix : Subsystem
  iy : Subsystem
  ix,iy : Outport
  wires:
  Mux/1 -> ix,iy/1
  ux,uy/1 -> Demux/1
  Demux/1 -> ix/1(ux)
  Demux/2 -> iy/1(uy)
  ix/1(ix) -> Mux/1
  iy/1(iy) -> Mux/2

== system MyModel_Open_v1_1/Drive & Motor/Subsystem/Six-phae PMSM/Source/abcxyz2qdz1z2/Clarke ==
  uab,ubc,uuv,uvw : Inport
  Demux : Demux
  Fcn1 : Fcn  Expr=(2*u[1]+u[2]+sqrt(3)*u[3])/6
  Fcn2 : Fcn  Expr=(sqrt(3)*u[2]+u[3]+2*u[4])/6
  Fcn6 : Fcn  Expr=(2*u[1]+u[2]-sqrt(3)*u[3])/6
  Fcn7 : Fcn  Expr=(-sqrt(3)*u[2]+u[3]+2*u[4])/6
  Mux1 : Mux  Inputs=2
  Mux2 : Mux
  Mux3 : Mux  Inputs=2
  ualpha,ubeta : Outport
  ux,uy : Outport  Port=2
  wires:
  Demux/2 -> Mux2/2
  Demux/3 -> Mux2/3
  Demux/4 -> Mux2/4
  Mux2/1 -> Fcn1/1, Fcn2/1, Fcn6/1, Fcn7/1
  uab,ubc,uuv,uvw/1 -> Demux/1
  Demux/1 -> Mux2/1
  Mux1/1 -> ualpha,ubeta/1
  Fcn1/1 -> Mux1/1
  Fcn2/1 -> Mux1/2
  Fcn6/1 -> Mux3/1
  Fcn7/1 -> Mux3/2
  Mux3/1 -> ux,uy/1

== system MyModel_Open_v1_1/Drive & Motor/Subsystem/Six-phae PMSM/Source/abcxyz2qdz1z2/PARK ==
  ualpha,ubeta : Inport
  s,c : Inport  Port=2
  Demux : Demux  Outputs=2
  Demux1 : Demux  Outputs=2
  Fcn : Fcn  Expr=u[1]*u[4]+u[2]*u[3]
  Fcn1 : Fcn  Expr=-u[1]*u[3]+u[2]*u[4]
  Mux : Mux
  Mux1 : Mux  Inputs=2
  ud,uq : Outport
  wires:
  Mux/1 -> Fcn/1, Fcn1/1
  s,c/1 -> Demux/1
  ualpha,ubeta/1 -> Demux1/1
  Demux1/1 -> Mux/1
  Demux1/2 -> Mux/2
  Demux/1 -> Mux/3
  Demux/2 -> Mux/4
  Fcn/1 -> Mux1/1
  Fcn1/1 -> Mux1/2
  Mux1/1 -> ud,uq/1

== system MyModel_Open_v1_1/Drive & Motor/Subsystem/Six-phae PMSM/Source/iq,id/id ==
  ud : Inport
  we : Inport  Port=2
  iq : Inport  Port=3
  1/Ld : Gain  Gain=1/Ld
  Lq/Ld : Gain  Gain=Lq/Ld
  Product : Product  RndMeth=Zero
  R/Ld : Gain  Gain=R/Ld
  Subtract : Sum  Inputs=-++
  d/dt(id) : Integrator
  id : Outport
  wires:
  d/dt(id)/1 -> id/1, R/Ld/1
  Subtract/1 -> d/dt(id)/1
  R/Ld/1 -> Subtract/1
  1/Ld/1 -> Subtract/2
  Lq/Ld/1 -> Subtract/3
  Product/1 -> Lq/Ld/1
  iq/1 -> Product/2
  we/1 -> Product/1
  ud/1 -> 1/Ld/1

== system MyModel_Open_v1_1/Drive & Motor/Subsystem/Six-phae PMSM/Source/iq,id/iq ==
  id : Inport
  we : Inport  Port=2
  uq : Inport  Port=3
  1/Lq : Gain  Gain=1/Lq
  Ld/Lq : Gain  Gain=Ld/Lq
  Product : Product  RndMeth=Zero
  R/Lq : Gain  Gain=R/Lq
  Subtract : Sum  Inputs=---+
  d/dt(iq) : Integrator
  flux/Lq : Gain  Gain=Flux/Lq
  iq : Outport
  wires:
  d/dt(iq)/1 -> iq/1, R/Lq/1
  Subtract/1 -> d/dt(iq)/1
  R/Lq/1 -> Subtract/1
  Ld/Lq/1 -> Subtract/2
  flux/Lq/1 -> Subtract/3
  1/Lq/1 -> Subtract/4
  uq/1 -> 1/Lq/1
  we/1 -> Product/2, flux/Lq/1
  id/1 -> Product/1
  Product/1 -> Ld/Lq/1

== system MyModel_Open_v1_1/Drive & Motor/Subsystem/Six-phae PMSM/Source/is/IClarke ==
  ialpha,ibeta : Inport
  ix,iy : Inport  Port=2
  Fcn1 : Fcn  Expr=u[1]+u[3]
  Fcn2 : Fcn  Expr=-1/2*u[1]+sqrt(3)/2*u[2]-1/2*u[3]-sqrt(3)/2*u[4]
  Fcn3 : Fcn  Expr=-sqrt(3)/2*u[1]+1/2*u[2]+sqrt(3)/2*u[3]+1/2*u[4]
  Fcn4 : Fcn  Expr=-u[2]-u[4]
  Fcn6 : Fcn  Expr=-1/2*u[1]-sqrt(3)/2*u[2]-1/2*u[3]+sqrt(3)/2*u[4]
  Fcn7 : Fcn  Expr=sqrt(3)/2*u[1]+1/2*u[2]-sqrt(3)/2*u[3]+1/2*u[4]
  Mux : Mux  Inputs=6
  Mux2 : Mux  Inputs=2
  iabcuvw : Outport
  wires:
  Mux2/1 -> Fcn1/1, Fcn2/1, Fcn6/1, Fcn7/1, Fcn4/1, Fcn3/1
  Fcn1/1 -> Mux/1
  Fcn2/1 -> Mux/2
  Fcn6/1 -> Mux/3
  Fcn7/1 -> Mux/4
  Fcn3/1 -> Mux/5
  Fcn4/1 -> Mux/6
  Mux/1 -> iabcuvw/1
  ialpha,ibeta/1 -> Mux2/1
  ix,iy/1 -> Mux2/2

== system MyModel_Open_v1_1/Drive & Motor/Subsystem/Six-phae PMSM/Source/is/IPARK ==
  s,c : Inport
  id,iq : Inport  Port=2
  Demux : Demux  Outputs=2
  Demux1 : Demux  Outputs=2
  Mux : Mux
  Mux1 : Mux  Inputs=2
  ialpha : Fcn  Expr=u[1]*u[4]-u[2]*u[3]
  ibeta : Fcn  Expr=u[1]*u[3]+u[2]*u[4]
  ialpha,ibeta : Outport
  wires:
  Mux/1 -> ibeta/1, ialpha/1
  Demux/2 -> Mux/2
  Demux/1 -> Mux/1
  id,iq/1 -> Demux/1
  Demux1/1 -> Mux/3
  Demux1/2 -> Mux/4
  s,c/1 -> Demux1/1
  ialpha/1 -> Mux1/1
  ibeta/1 -> Mux1/2
  Mux1/1 -> ialpha,ibeta/1

== system MyModel_Open_v1_1/Drive & Motor/Subsystem/Six-phae PMSM/Source/ix,iy/ix ==
  ux : Inport
  1/Lz : Gain  Gain=1/Lz
  R/Lz : Gain  Gain=R/Lz
  Subtract : Sum  Inputs=-+
  d/dt(ix) : Integrator
  ix : Outport
  wires:
  d/dt(ix)/1 -> ix/1, R/Lz/1
  Subtract/1 -> d/dt(ix)/1
  R/Lz/1 -> Subtract/1
  1/Lz/1 -> Subtract/2
  ux/1 -> 1/Lz/1

== system MyModel_Open_v1_1/Drive & Motor/Subsystem/Six-phae PMSM/Source/ix,iy/iy ==
  uy : Inport
  1/Lz : Gain  Gain=1/Lz
  R/Lz : Gain  Gain=R/Lz
  Subtract : Sum  Inputs=-+
  d/dt(iy) : Integrator
  iy : Outport
  wires:
  d/dt(iy)/1 -> iy/1, R/Lz/1
  Subtract/1 -> d/dt(iy)/1
  R/Lz/1 -> Subtract/1
  1/Lz/1 -> Subtract/2
  uy/1 -> 1/Lz/1

== matlab function MyModel_Open_v1_1/Drive & Motor/Subsystem/MATLAB Function ==
  data: u input; y output
function y = fcn(u)

y = 30 * u / pi;

== matlab function MyModel_Open_v1_1/Drive & Motor/Embedded MATLAB Function ==
  data: uo output; uab input; ua output; ubc input; ucd input; ude input; uef input; ub output; uc output; ud output; ue output; uf output
function [uo,ua,ub,uc,ud,ue,uf] = fcn(uab,ubc,ucd,ude,uef)

%#codegen
uxx = [uab,ubc,ucd,ude,uef,0,0]';
T = [0 1 -1 0 0 0 0;
     0 0 1 -1 0 0 0;
     1 0 0 1 -1 0 0;
     0 0 0 0 1 -1 0;
     0 0 0 0 0 1 -1;
     0 1 1 1 0 0 0;
     0 0 0 0 1 1 1];
I = T \ uxx;
uo = I(1);
ua = I(2);
ub = I(3);
uc = I(4);
ud = I(5);
ue = I(6);
uf = I(7);

== matlab function MyModel_Open_v1_1/Drive & Motor/Embedded MATLAB Function1 ==
  data: uo output; uab input; ua output; ubc input; ucd input; ude input; uef input; ub output; uc output; ud output; ue output; uf output
function [uo,ua,ub,uc,ud,ue,uf] = fcn(uab,ubc,ucd,ude,uef)

%#codegen
uxx = [uab,ubc,ucd,ude,uef,0,0]';
T = [0 1 -1 0 0 0 0;
     0 0 1 -1 0 0 0;
     1 0 0 1 -1 0 0;
     0 0 0 0 1 -1 0;
     0 0 0 0 0 1 -1;
     0 1 1 1 0 0 0;
     0 0 0 0 1 1 1];
I = T \ uxx;
uo = I(1);
ua = I(2);
ub = I(3);
uc = I(4);
ud = I(5);
ue = I(6);
uf = I(7);

== matlab function MyModel_Open_v1_1/Drive & Motor/clark1 ==
  data: falpha output; fa input; fbeta output; fb input; fc input; fd input; fe input; fx output; fy output; fo1 output; fo2 output; ff input
function [falpha,fbeta,fx,fy,fo1,fo2] = clark(fa,fb,fc,fd,fe,ff)

T=1/sqrt(3)*[1,  (-1/2),    (-1/2),       sqrt(3)/2,  -sqrt(3)/2,  0;
       0,  sqrt(3)/2, (-sqrt(3)/2), 1/2,        1/2,        -1;
       1,  (-1/2),    (-1/2),       -sqrt(3)/2, sqrt(3)/2,   0;
       0,  -sqrt(3)/2,sqrt(3)/2,    1/2,        1/2,        -1;
       1,  1,         1,            0,          0,           0;
       0,  0,         0,            1,          1,           1];
X=[fa;fb;fc;fd;fe;ff];
Y=T*X;
falpha=Y(1);
fbeta=Y(2);
fx=Y(3);
fy=Y(4);
fo1=Y(5);
fo2=Y(6);
end

== matlab function MyModel_Open_v1_1/SVPWM2/Embedded MATLAB Function2 ==
  data: N input; t1 output; Ualpha input; Ubeta input; Tpwm input; t2 output; t3 output; t4 output; t0 output; udc input; Ux input; Uy input; t1cp output; t2cp output; t3cp output; t4cp output
function [t1, t2, t3, t4, t0, t1cp, t2cp, t3cp, t4cp] = fcn(N, Ualpha, Ubeta, Tpwm, udc, Ux,Uy)

m=sqrt(3)/2+1/2*1i;

%等功率clarke反变换
ab44=1/sqrt(3)*udc*[1,m^4,m^8,m,m^5,m^9]*[1;0;0;1;0;0];
xy44=1/sqrt(3)*udc*[1,m^8,m^4,m^5,m,m^9]*[1;0;0;1;0;0];

ab64=1/sqrt(3)*udc*[1,m^4,m^8,m,m^5,m^9]*[1;1;0;1;0;0];
xy64=1/sqrt(3)*udc*[1,m^8,m^4,m^5,m,m^9]*[1;1;0;1;0;0];
        
ab66=1/sqrt(3)*udc*[1,m^4,m^8,m,m^5,m^9]*[1;1;0;1;1;0];
xy66=1/sqrt(3)*udc*[1,m^8,m^4,m^5,m,m^9]*[1;1;0;1;1;0];

ab26=1/sqrt(3)*udc*[1,m^4,m^8,m,m^5,m^9]*[0;1;0;1;1;0];
xy26=1/sqrt(3)*udc*[1,m^8,m^4,m^5,m,m^9]*[0;1;0;1;1;0];

ab22=1/sqrt(3)*udc*[1,m^4,m^8,m,m^5,m^9]*[0;1;0;0;1;0];
xy22=1/sqrt(3)*udc*[1,m^8,m^4,m^5,m,m^9]*[0;1;0;0;1;0];

ab32=1/sqrt(3)*udc*[1,m^4,m^8,m,m^5,m^9]*[0;1;1;0;1;0];
xy32=1/sqrt(3)*udc*[1,m^8,m^4,m^5,m,m^9]*[0;1;1;0;1;0];

ab33=1/sqrt(3)*udc*[1,m^4,m^8,m,m^5,m^9]*[0;1;1;0;1;1];
xy33=1/sqrt(3)*udc*[1,m^8,m^4,m^5,m,m^9]*[0;1;1;0;1;1];

ab13=1/sqrt(3)*udc*[1,m^4,m^8,m,m^5,m^9]*[0;0;1;0;1;1];
xy13=1/sqrt(3)*udc*[1,m^8,m^4,m^5,m,m^9]*[0;0;1;0;1;1];

ab11=1/sqrt(3)*udc*[1,m^4,m^8,m,m^5,m^9]*[0;0;1;0;0;1];
xy11=1/sqrt(3)*udc*[1,m^8,m^4,m^5,m,m^9]*[0;0;1;0;0;1];

ab51=1/sqrt(3)*udc*[1,m^4,m^8,m,m^5,m^9]*[1;0;1;0;0;1];
xy51=1/sqrt(3)*udc*[1,m^8,m^4,m^5,m,m^9]*[1;0;1;0;0;1];

ab55=1/sqrt(3)*udc*[1,m^4,m^8,m,m^5,m^9]*[1;0;1;1;0;1];
xy55=1/sqrt(3)*udc*[1,m^8,m^4,m^5,m,m^9]*[1;0;1;1;0;1];

ab45=1/sqrt(3)*udc*[1,m^4,m^8,m,m^5,m^9]*[1;0;0;1;0;1];
xy45=1/sqrt(3)*udc*[1,m^8,m^4,m^5,m,m^9]*[1;0;0;1;0;1];

switch N
    case 1
        X=[real(ab55),real(ab45),real(ab44),real(ab64);
           imag(ab55),imag(ab45),imag(ab44),imag(ab64);
           real(xy55),real(xy45),real(xy44),real(xy64);
           imag(xy55),imag(xy45),imag(xy44),imag(xy64)];

    case 2
        X=[real(ab45),real(ab44),real(ab64),real(ab66);
           imag(ab45),imag(ab44),imag(ab64),imag(ab66);
           real(xy45),real(xy44),real(xy64),real(xy66);
           imag(xy45),imag(xy44),imag(xy64),imag(xy66)];

    case 3
        X=[real(ab44),real(ab64),real(ab66),real(ab26);
           imag(ab44),imag(ab64),imag(ab66),imag(ab26);
           real(xy44),real(xy64),real(xy66),real(xy26);
           imag(xy44),imag(xy64),imag(xy66),imag(xy26)];

    case 4
        X=[real(ab64),real(ab66),real(ab26),real(ab22);
           imag(ab64),imag(ab66),imag(ab26),imag(ab22);
           real(xy64),real(xy66),real(xy26),real(xy22);
           imag(xy64),imag(xy66),imag(xy26),imag(xy22)];

    case 5
        X=[real(ab66),real(ab26),real(ab22),real(ab32);
           imag(ab66),imag(ab26),imag(ab22),imag(ab32);
           real(xy66),real(xy26),real(xy22),real(xy32);
           imag(xy66),imag(xy26),imag(xy22),imag(xy32)];

    case 6
        X=[real(ab26),real(ab22),real(ab32),real(ab33);
           imag(ab26),imag(ab22),imag(ab32),imag(ab33);
           real(xy26),real(xy22),real(xy32),real(xy33);
           imag(xy26),imag(xy22),imag(xy32),imag(xy33)];

    case 7
        X=[real(ab22),real(ab32),real(ab33),real(ab13);
           imag(ab22),imag(ab32),imag(ab33),imag(ab13);
           real(xy22),real(xy32),real(xy33),real(xy13);
           imag(xy22),imag(xy32),imag(xy33),imag(xy13)];

    case 8
        X=[real(ab32),real(ab33),real(ab13),real(ab11);
           imag(ab32),imag(ab33),imag(ab13),imag(ab11);
           real(xy32),real(xy33),real(xy13),real(xy11);
           imag(xy32),imag(xy33),imag(xy13),imag(xy11)];

    case 9
        X=[real(ab33),real(ab13),real(ab11),real(ab51);
           imag(ab33),imag(ab13),imag(ab11),imag(ab51);
           real(xy33),real(xy13),real(xy11),real(xy51);
           imag(xy33),imag(xy13),imag(xy11),imag(xy51)];

    case 10
        X=[real(ab13),real(ab11),real(ab51),real(ab55);
           imag(ab13),imag(ab11),imag(ab51),imag(ab55);
           real(xy13),real(xy11),real(xy51),real(xy55);
           imag(xy13),imag(xy11),imag(xy51),imag(xy55)];

    case 11
        X=[real(ab11),real(ab51),real(ab55),real(ab45);
           imag(ab11),imag(ab51),imag(ab55),imag(ab45);
           real(xy11),real(xy51),real(xy55),real(xy45);
           imag(xy11),imag(xy51),imag(xy55),imag(xy45)];

    case 12
        X=[real(ab51),real(ab55),real(ab45),real(ab44);
           imag(ab51),imag(ab55),imag(ab45),imag(ab44);
           real(xy51),real(xy55),real(xy45),real(xy44);
           imag(xy51),imag(xy55),imag(xy45),imag(xy44)];

    otherwise
        X=[0,0,0,0;
           0,0,0,0;
           0,0,0,0;
           0,0,0,0];

end
Y=[Ualpha;Ubeta;Ux;Uy]*Tpwm;
T = X \ Y;

% t1=T(1);
% if t1<1e-6
%     t1=1e-6;
% end
% t2=T(2);
% if t2<1e-6
%     t2=1e-6;
% end
% t3=T(3);
% if t3<1e-6
%     t3=1e-6;
% end
% t4=T(4);
% if t4<1e-6
%     t4=1e-6;
% end

% T1=T(1);
% T2=T(2);
% T3=T(3);
% T4=T(4);

t1cp = 0;
t2cp = 0;
t3cp = 0;
t4cp = 0;

if T(1) >= 0
    t1 = T(1);
else
    t1 = 0;
    t1cp = -T(1);
end
if T(2) >= 0
    t2 = T(2);
else
    t2 = 0;
    t2cp = -T(2);
end
if T(3) >= 0
    t3 = T(3);
else
    t3 = 0;
    t3cp = -T(3);
end
if T(4) >= 0
    t4 = T(4);
else
    t4 = 0;
    t4cp = -T(4);
end

Tsum=t1+t2+t3+t4;
if Tsum>Tpwm
    t1=t1*Tpwm/Tsum;
    t2=t2*Tpwm/Tsum;
    t3=t3*Tpwm/Tsum;
    t4=t4*Tpwm/Tsum;
end
t0=Tpwm-t1-t2-t3-t4;
end

== matlab function MyModel_Open_v1_1/SVPWM2/Embedded MATLAB Function6 ==
  data: N output; ualfa input; ubeta input; TH output
function [N,TH] = fcn(ualfa,ubeta)

%#xsxx
[TH,~] = cart2pol(ualfa,ubeta);
if TH<0
    TH=TH+2*pi;
end
N=floor((TH+pi/12)/(pi/6))+1;
if N==13
    N=1;
end

== matlab function MyModel_Open_v1_1/SVPWM2/rest of others ==
  data: N input; T1 input; T2 input; T3 input; T4 input; T0 input; a1 output; a2 output; b1 output; b2 output; c1 output; c2 output; d1 output; d2 output; e1 output; e2 output; f1 output; f2 output; t1cp input; t2cp input; t3cp input; t4cp input
function [a1,a2,b1,b2,c1,c2,d1,d2,e1,e2,f1,f2] = fcn(N,T1,T2,T3,T4,T0,t1cp,t2cp,t3cp,t4cp)

%#xsxx
Ta=T0/4;
Tb=Ta+T2;
Tc=Tb+T1;
Td=Tc+T0/2;
Te=Td+T4;
Tf=Te+T3;

Ta1=T0/4;
Tb1=Ta1+T1;
Tc1=Tb1+T2;
Td1=Tc1+T0/2;
Te1=Td1+T3;
Tf1=Te1+T4;

%a1:phase A CMPA
%a2:phase A CMPB

a1 = 0;
a2 = 0;
b1 = 0;
b2 = 0;
c1 = 0;
c2 = 0;
d1 = 0;
d2 = 0;
e1 = 0;
e2 = 0;
f1 = 0;
f2 = 0;

if N==1
    a1=Ta;%TIme of "00" voltage vector 
    a2=Tf;%TIme of "48" voltage vector 
    d1=Ta;
    d2=Tf;
    b1=Tc;%TIme of "51" voltage vector 
    b2=Te + t1cp + t2cp + t3cp;%TIme of "56" voltage vector 
    e1=Tc;
    e2=Td + t1cp +t2cp +t3cp + t4cp;
    c1=Tb;%TIme of "49" voltage vector 
    c2=Td + t2cp + t3cp + t4cp;%TIme of "63" voltage vector 
    f1=Ta;
    f2=Td + t3cp + t4cp;
elseif N==2
    a1=Ta;
    a2=Tf;
    d1=Ta;
    d2=Tf;
    b1=Tc;
    b2=Tf + t1cp + t2cp;
    e1=Tc;
    e2=Te + t1cp + t2cp + t3cp;
    c1=Tc;
    c2=Td + t1cp + t2cp + t3cp + t4cp;
    f1=Tb;
    f2=Td + t2cp + t3cp + t4cp;
elseif N==3
    a1=Ta1;
    a2=Te1 + t4cp;
    d1=Ta1;
    d2=Tf1;
    b1=Tb1;
    b2=Tf1 + t1cp;
    e1=Tc1;
    e2=Tf1 + t1cp + t2cp;
    c1=Tc1;
    c2=Td1 + t1cp + t2cp + t3cp + t4cp;
    f1=Tc1;
    f2=Td1 + t1cp + t2cp + t3cp + t4cp;
elseif N==4
    a1=Ta1;
    a2=Td1 + t3cp + t4cp;
    d1=Ta1;
    d2=Te1 + t4cp;
    b1=Ta1;
    b2=Tf1;
    e1=Tb1;
    e2=Tf1 + t1cp;
    c1=Tc1;
    c2=Td1 + t1cp + t2cp + t3cp + t4cp;
    f1=Tc1;
    f2=Td1 + t1cp + t2cp + t3cp + t4cp;
elseif N==5
    a1=Tb;
    a2=Td + t2cp + t3cp + t4cp;
    d1=Ta;
    d2=Td + t3cp + t4cp;
    b1=Ta;
    b2=Tf;
    e1=Ta;
    e2=Tf;
    c1=Tc;
    c2=Te + t1cp + t2cp + t3cp;
    f1=Tc;
    f2=Td + t1cp + t2cp + t3cp + t4cp;
elseif N==6
    a1=Tc;
    a2=Td + t1cp + t2cp + t3cp + t4cp;
    d1=Tb;
    d2=Td + t2cp + t3cp + t4cp;
    b1=Ta;
    b2=Tf;
    e1=Ta;
    e2=Tf;
    c1=Tc;
    c2=Tf + t1cp + t2cp;
    f1=Tc;
    f2=Te + t1cp + t2cp + t3cp;
elseif N==7
    a1=Tc1;
    a2=Td1 + t1cp + t2cp + t3cp + t4cp;
    d1=Tc1;
    d2=Td1 + t1cp + t2cp + t3cp + t4cp;
    b1=Ta1;
    b2=Te1 + t4cp;
    e1=Ta1;
    e2=Tf1;
    c1=Tb1;
    c2=Tf1 + t1cp;
    f1=Tc1;
    f2=Tf1 + t1cp + t2cp;
elseif N==8
    a1=Tc1;
    a2=Td1 + t1cp + t2cp + t3cp + t4cp;
    d1=Tc1;
    d2=Td1 + t1cp + t2cp + t3cp + t4cp;
    b1=Ta1;
    b2=Td1 + t3cp + t4cp;
    e1=Ta1;
    e2=Te1 + t4cp;
    c1=Ta1;
    c2=Tf1;
    f1=Tb1;
    f2=Tf1 + t1cp;
elseif N==9
    a1=Tc;
    a2=Te + t1cp + t2cp + t3cp;
    d1=Tc;
    d2=Td + t1cp + t2cp + t3cp + t4cp;
    b1=Tb;
    b2=Td + t2cp + t3cp + t4cp;
    e1=Ta;
    e2=Td + t3cp + t4cp;
    c1=Ta;
    c2=Tf;
    f1=Ta;
    f2=Tf;
elseif N==10
    a1=Tc;
    a2=Tf + t1cp + t2cp;
    d1=Tc;
    d2=Te + t1cp + t2cp + t3cp;
    b1=Tc;
    b2=Td + t1cp + t2cp + t3cp + t4cp;
    e1=Tb;
    e2=Td + t2cp + t3cp + t4cp;
    c1=Ta;
    c2=Tf;
    f1=Ta;
    f2=Tf;
elseif N==11
    a1=Tb1;
    a2=Tf1 + t1cp;
    d1=Tc1;
    d2=Tf1 + t1cp + t2cp;
    b1=Tc1;
    b2=Td1 + t1cp + t2cp + t3cp + t4cp;
    e1=Tc1;
    e2=Td1 + t1cp + t2cp + t3cp + t4cp;
    c1=Ta1;
    c2=Te1 + t4cp;
    f1=Ta1;
    f2=Tf1;
elseif N==12
    a1=Ta1;
    a2=Tf1;
    d1=Tb1;
    d2=Tf1 + t1cp;
    b1=Tc1;
    b2=Td1 + t1cp + t2cp + t3cp + t4cp;
    e1=Tc1;
    e2=Td1 + t1cp + t2cp + t3cp + t4cp;
    c1=Ta1;
    c2=Td1 + t3cp + t4cp;
    f1=Ta1;
    f2=Te1 + t4cp;
end
